simulink model "Block-Diagram-1"  (R2023b)
settings: Solver=VariableStepAuto  StartTime=0.0  StopTime=10.0  RelTol=1e-3
values from neighbouring files (symbols this model uses):
  G1_den = [1 0 0]    [Block_Diagram_2.m]    (also in CSE_Lab3_BlockDiagram1.m)
  G1_num = [1]    [Block_Diagram_2.m]    (also in CSE_Lab3_BlockDiagram1.m = 1)
  G2_den = [1 1]    [Block_Diagram_2.m]    (also in CSE_Lab3_BlockDiagram1.m)
  G2_num = [1]    [Block_Diagram_2.m]    (also in CSE_Lab3_BlockDiagram1.m = 1)
  G3_den = [1 0]    [Block_Diagram_2.m]    (also in CSE_Lab3_BlockDiagram1.m)
  G3_num = [1]    [Block_Diagram_2.m]    (also in CSE_Lab3_BlockDiagram1.m = 1)
  H1_den = [1 0]    [Block_Diagram_2.m]    (also in CSE_Lab3_BlockDiagram1.m)
  H1_num = [1]    [Block_Diagram_2.m]    (also in CSE_Lab3_BlockDiagram1.m = 1)
  H2_den = [1 -1]    [Block_Diagram_2.m]    (also in CSE_Lab3_BlockDiagram1.m)
  H2_num = [1]    [Block_Diagram_2.m]    (also in CSE_Lab3_BlockDiagram1.m = 1)
  H3_den = [1 -2]    [Block_Diagram_2.m]    (also in CSE_Lab3_BlockDiagram1.m)
  H3_num = [1]    [Block_Diagram_2.m]    (also in CSE_Lab3_BlockDiagram1.m = 1)
undefined symbols (not defined in the file or in its folder): TF_den, TF_num
settings Model: Creator=Ariane Mae Umali  LastModifiedBy=Ariane Mae Umali

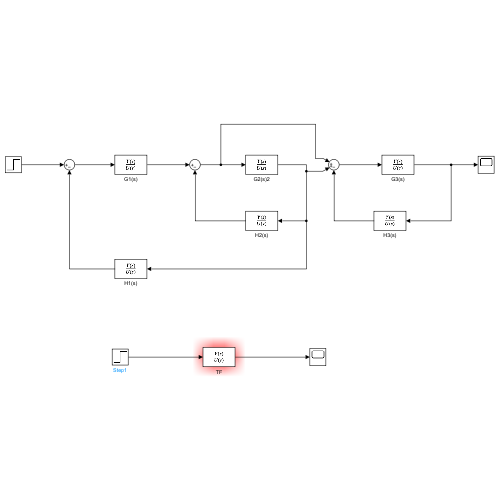
[thumbnail: Simulink's stored preview of the top-level diagram]
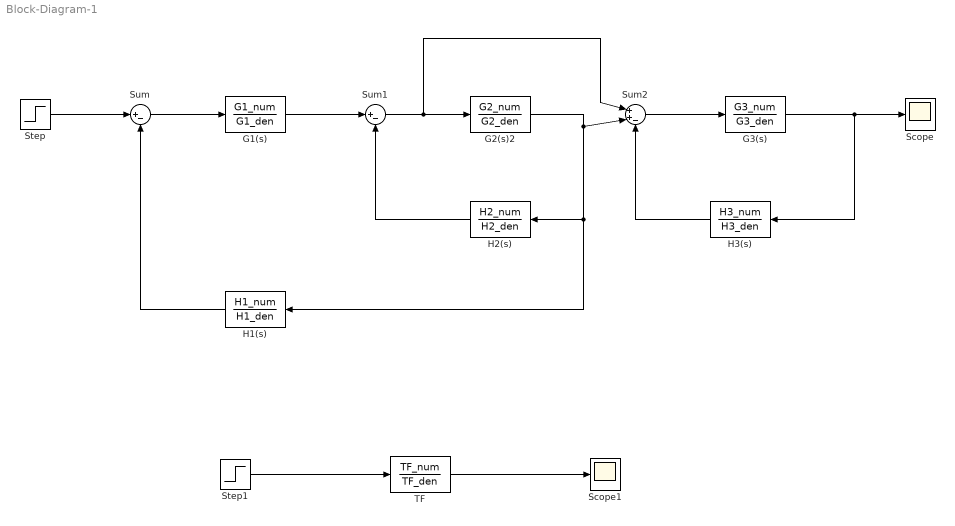
== system Block-Diagram-1 ==
  G1(s) : TransferFcn  Numerator=G1_num  Denominator=G1_den
  G2(s)2 : TransferFcn  Numerator=G2_num  Denominator=G2_den
  G3(s) : TransferFcn  Numerator=G3_num  Denominator=G3_den
  H1(s) : TransferFcn  Numerator=H1_num  Denominator=H1_den
  H2(s) : TransferFcn  Numerator=H2_num  Denominator=H2_den
  H3(s) : TransferFcn  Numerator=H3_num  Denominator=H3_den
  Scope : Scope
  Scope1 : Scope
  Step : Step  SampleTime=0
  Step1 : Step  SampleTime=0
  Sum : Sum  Inputs=|+-
  Sum1 : Sum  Inputs=|+-
  Sum2 : Sum  Inputs=|++-
  TF : TransferFcn  Numerator=TF_num  Denominator=TF_den
  wires:
  Step/1 -> Sum/1
  Sum/1 -> G1(s)/1
  G1(s)/1 -> Sum1/1
  Sum1/1 -> Sum2/1, G2(s)2/1
  Sum2/1 -> G3(s)/1
  G3(s)/1 -> H3(s)/1, Scope/1
  H3(s)/1 -> Sum2/3
  G2(s)2/1 -> H1(s)/1, H2(s)/1, Sum2/2
  H2(s)/1 -> Sum1/2
  H1(s)/1 -> Sum/2
  Step1/1 -> TF/1
  TF/1 -> Scope1/1
